simulink model "DriveSystemControl"  (R2023b)
settings: Solver=FixedStepAuto  StartTime=0.0  StopTime=Inf  FixedStep=0.001  RelTol=1e-3
PostLoadFcn:
  | if any(exist('dsrtsu_mdlpostloadfcn', 'file') ~= 0), dsrtsu_mdlpostloadfcn('Execute', bdroot); end
InitFcn:
  | , if any(exist('rtifpga_mdlclblib', 'file') ~= 0), rtifpga_mdlclblib('Init', bdroot); end,
  | , if any(exist('dsmpb_private', 'file') ~= 0), dsmpb_private('dsmpb_mdlclblib', 'Init', bdroot); end,
libraries: dsmpblib x2
(part 3 of 11)

== system DriveSystemControl/Bus Configuration (1) - In/Manipulation/Virya Controller CAN File 08082024/WIP/CANChannel/PDUs/MainController/notUsed ==
  Feature Switch : Subsystem
  ISignal Overwrite Value : Subsystem
  _notUsed_ : BusCreator  Inputs=2
  notUsed : Outport
  wires:
  _notUsed_/1 -> notUsed/1  "notUsed"
  Feature Switch/1(Feature Switch) -> _notUsed_/1  "Feature Switch"
  ISignal Overwrite Value/1(ISignal Overwrite Value) -> _notUsed_/2  "ISignal Overwrite Value"

== system DriveSystemControl/Bus Configuration (1) - In/Manipulation/Virya Controller CAN File 08082024/WIP/CANChannel/PDUs/MainController/setAutoParkBreak ==
  Feature Switch : Subsystem
  ISignal Overwrite Value : Subsystem
  _setAutoParkBreak_ : BusCreator  Inputs=2
  setAutoParkBreak : Outport
  wires:
  _setAutoParkBreak_/1 -> setAutoParkBreak/1  "setAutoParkBreak"
  Feature Switch/1(Feature Switch) -> _setAutoParkBreak_/1  "Feature Switch"
  ISignal Overwrite Value/1(ISignal Overwrite Value) -> _setAutoParkBreak_/2  "ISignal Overwrite Value"

== system DriveSystemControl/Bus Configuration (1) - In/Manipulation/Virya Controller CAN File 08082024/WIP/CANChannel/PDUs/MainController/setBreake ==
  Feature Switch : Subsystem
  ISignal Overwrite Value : Subsystem
  _setBreake_ : BusCreator  Inputs=2
  setBreake : Outport
  wires:
  _setBreake_/1 -> setBreake/1  "setBreake"
  Feature Switch/1(Feature Switch) -> _setBreake_/1  "Feature Switch"
  ISignal Overwrite Value/1(ISignal Overwrite Value) -> _setBreake_/2  "ISignal Overwrite Value"

== system DriveSystemControl/Bus Configuration (1) - In/Manipulation/Virya Controller CAN File 08082024/WIP/CANChannel/PDUs/MainController/setDirection ==
  Feature Switch : Subsystem
  ISignal Overwrite Value : Subsystem
  _setDirection_ : BusCreator  Inputs=2
  setDirection : Outport
  wires:
  _setDirection_/1 -> setDirection/1  "setDirection"
  Feature Switch/1(Feature Switch) -> _setDirection_/1  "Feature Switch"
  ISignal Overwrite Value/1(ISignal Overwrite Value) -> _setDirection_/2  "ISignal Overwrite Value"

== system DriveSystemControl/Bus Configuration (1) - In/Manipulation/Virya Controller CAN File 08082024/WIP/CANChannel/PDUs/MainController/setDriveMode ==
  Feature Switch : Subsystem
  ISignal Overwrite Value : Subsystem
  _setDriveMode_ : BusCreator  Inputs=2
  setDriveMode : Outport
  wires:
  _setDriveMode_/1 -> setDriveMode/1  "setDriveMode"
  Feature Switch/1(Feature Switch) -> _setDriveMode_/1  "Feature Switch"
  ISignal Overwrite Value/1(ISignal Overwrite Value) -> _setDriveMode_/2  "ISignal Overwrite Value"

== system DriveSystemControl/Bus Configuration (1) - In/Manipulation/Virya Controller CAN File 08082024/WIP/CANChannel/PDUs/MainController/setVelocity ==
  Feature Switch : Subsystem
  ISignal Overwrite Value : Subsystem
  _setVelocity_ : BusCreator  Inputs=2
  setVelocity : Outport
  wires:
  _setVelocity_/1 -> setVelocity/1  "setVelocity"
  Feature Switch/1(Feature Switch) -> _setVelocity_/1  "Feature Switch"
  ISignal Overwrite Value/1(ISignal Overwrite Value) -> _setVelocity_/2  "ISignal Overwrite Value"

== system DriveSystemControl/Bus Configuration (1) - In/Manipulation/Virya Controller CAN File 08082024/WIP/CANChannel/PDUs/MainController/steeringPower ==
  Feature Switch : Subsystem
  ISignal Overwrite Value : Subsystem
  _steeringPower_ : BusCreator  Inputs=2
  steeringPower : Outport
  wires:
  _steeringPower_/1 -> steeringPower/1  "steeringPower"
  Feature Switch/1(Feature Switch) -> _steeringPower_/1  "Feature Switch"
  ISignal Overwrite Value/1(ISignal Overwrite Value) -> _steeringPower_/2  "ISignal Overwrite Value"

== system DriveSystemControl/Bus Configuration (1) - In/Manipulation/Virya Controller CAN File 08082024/WIP/CANChannel/PDUs/TCU01/sigBrake ==
  Feature Switch : Subsystem
  ISignal Overwrite Value : Subsystem
  _sigBrake_ : BusCreator  Inputs=2
  sigBrake : Outport
  wires:
  _sigBrake_/1 -> sigBrake/1  "sigBrake"
  Feature Switch/1(Feature Switch) -> _sigBrake_/1  "Feature Switch"
  ISignal Overwrite Value/1(ISignal Overwrite Value) -> _sigBrake_/2  "ISignal Overwrite Value"

== system DriveSystemControl/Bus Configuration (1) - In/Manipulation/Virya Controller CAN File 08082024/WIP/CANChannel/PDUs/TCU01/sigControllerTemperature ==
  Feature Switch : Subsystem
  ISignal Overwrite Value : Subsystem
  _sigControllerTemperature_ : BusCreator  Inputs=2
  sigControllerTemperature : Outport
  wires:
  _sigControllerTemperature_/1 -> sigControllerTemperature/1  "sigControllerTemperature"
  Feature Switch/1(Feature Switch) -> _sigControllerTemperature_/1  "Feature Switch"
  ISignal Overwrite Value/1(ISignal Overwrite Value) -> _sigControllerTemperature_/2  "ISignal Overwrite Value"

== system DriveSystemControl/Bus Configuration (1) - In/Manipulation/Virya Controller CAN File 08082024/WIP/CANChannel/PDUs/TCU01/sigDriveMode ==
  Feature Switch : Subsystem
  ISignal Overwrite Value : Subsystem
  _sigDriveMode_ : BusCreator  Inputs=2
  sigDriveMode : Outport
  wires:
  _sigDriveMode_/1 -> sigDriveMode/1  "sigDriveMode"
  Feature Switch/1(Feature Switch) -> _sigDriveMode_/1  "Feature Switch"
  ISignal Overwrite Value/1(ISignal Overwrite Value) -> _sigDriveMode_/2  "ISignal Overwrite Value"

== system DriveSystemControl/Bus Configuration (1) - In/Manipulation/Virya Controller CAN File 08082024/WIP/CANChannel/PDUs/TCU01/sigMotorTemperature ==
  Feature Switch : Subsystem
  ISignal Overwrite Value : Subsystem
  _sigMotorTemperature_ : BusCreator  Inputs=2
  sigMotorTemperature : Outport
  wires:
  _sigMotorTemperature_/1 -> sigMotorTemperature/1  "sigMotorTemperature"
  Feature Switch/1(Feature Switch) -> _sigMotorTemperature_/1  "Feature Switch"
  ISignal Overwrite Value/1(ISignal Overwrite Value) -> _sigMotorTemperature_/2  "ISignal Overwrite Value"

== system DriveSystemControl/Bus Configuration (1) - In/Manipulation/Virya Controller CAN File 08082024/WIP/CANChannel/PDUs/TCU01/sigRMSCurrent ==
  Feature Switch : Subsystem
  ISignal Overwrite Value : Subsystem
  _sigRMSCurrent_ : BusCreator  Inputs=2
  sigRMSCurrent : Outport
  wires:
  _sigRMSCurrent_/1 -> sigRMSCurrent/1  "sigRMSCurrent"
  Feature Switch/1(Feature Switch) -> _sigRMSCurrent_/1  "Feature Switch"
  ISignal Overwrite Value/1(ISignal Overwrite Value) -> _sigRMSCurrent_/2  "ISignal Overwrite Value"

== system DriveSystemControl/Bus Configuration (1) - In/Manipulation/Virya Controller CAN File 08082024/WIP/CANChannel/PDUs/TCU01/sigSpeed ==
  Feature Switch : Subsystem
  ISignal Overwrite Value : Subsystem
  _sigSpeed_ : BusCreator  Inputs=2
  sigSpeed : Outport
  wires:
  _sigSpeed_/1 -> sigSpeed/1  "sigSpeed"
  Feature Switch/1(Feature Switch) -> _sigSpeed_/1  "Feature Switch"
  ISignal Overwrite Value/1(ISignal Overwrite Value) -> _sigSpeed_/2  "ISignal Overwrite Value"

== system DriveSystemControl/Bus Configuration (1) - In/Manipulation/Virya Controller CAN File 08082024/WIP/CANChannel/PDUs/TCU01/sigThrottle ==
  Feature Switch : Subsystem
  ISignal Overwrite Value : Subsystem
  _sigThrottle_ : BusCreator  Inputs=2
  sigThrottle : Outport
  wires:
  _sigThrottle_/1 -> sigThrottle/1  "sigThrottle"
  Feature Switch/1(Feature Switch) -> _sigThrottle_/1  "Feature Switch"
  ISignal Overwrite Value/1(ISignal Overwrite Value) -> _sigThrottle_/2  "ISignal Overwrite Value"

== system DriveSystemControl/Bus Configuration (1) - In/Manipulation/Virya Controller CAN File 08082024/WIP/CANChannel/PDUs/TCU02/sigCapacitorVoltage ==
  Feature Switch : Subsystem
  ISignal Overwrite Value : Subsystem
  _sigCapacitorVoltage_ : BusCreator  Inputs=2
  sigCapacitorVoltage : Outport
  wires:
  _sigCapacitorVoltage_/1 -> sigCapacitorVoltage/1  "sigCapacitorVoltage"
  Feature Switch/1(Feature Switch) -> _sigCapacitorVoltage_/1  "Feature Switch"
  ISignal Overwrite Value/1(ISignal Overwrite Value) -> _sigCapacitorVoltage_/2  "ISignal Overwrite Value"

== system DriveSystemControl/Bus Configuration (1) - In/Manipulation/Virya Controller CAN File 08082024/WIP/CANChannel/PDUs/TCU02/sigMotorRPM ==
  Feature Switch : Subsystem
  ISignal Overwrite Value : Subsystem
  _sigMotorRPM_ : BusCreator  Inputs=2
  sigMotorRPM : Outport
  wires:
  _sigMotorRPM_/1 -> sigMotorRPM/1  "sigMotorRPM"
  Feature Switch/1(Feature Switch) -> _sigMotorRPM_/1  "Feature Switch"
  ISignal Overwrite Value/1(ISignal Overwrite Value) -> _sigMotorRPM_/2  "ISignal Overwrite Value"

== system DriveSystemControl/Bus Configuration (1) - In/Manipulation/Virya Controller CAN File 08082024/WIP/CANChannel/PDUs/TCU02/sigOdometer ==
  Feature Switch : Subsystem
  ISignal Overwrite Value : Subsystem
  _sigOdometer_ : BusCreator  Inputs=2
  sigOdometer : Outport
  wires:
  _sigOdometer_/1 -> sigOdometer/1  "sigOdometer"
  Feature Switch/1(Feature Switch) -> _sigOdometer_/1  "Feature Switch"
  ISignal Overwrite Value/1(ISignal Overwrite Value) -> _sigOdometer_/2  "ISignal Overwrite Value"

== system DriveSystemControl/Bus Configuration (1) - In/Manipulation/Virya Controller CAN File 08082024/WIP/CANChannel/PDUs/TCU03/Controller_CompleteFaults ==
  Feature Switch : Subsystem
  ISignal Overwrite Value : Subsystem
  _Controller_CompleteFaults_ : BusCreator  Inputs=2
  Controller_CompleteFaults : Outport
  wires:
  _Controller_CompleteFaults_/1 -> Controller_CompleteFaults/1  "Controller_CompleteFaults"
  Feature Switch/1(Feature Switch) -> _Controller_CompleteFaults_/1  "Feature Switch"
  ISignal Overwrite Value/1(ISignal Overwrite Value) -> _Controller_CompleteFaults_/2  "ISignal Overwrite Value"

== system DriveSystemControl/Bus Configuration (1) - In/Manipulation/Virya Controller CAN File 08082024/WIP/CANChannel/PDUs/TCU03/sig5VSupplyFailure ==
  Feature Switch : Subsystem
  ISignal Overwrite Value : Subsystem
  _sig5VSupplyFailure_ : BusCreator  Inputs=2
  sig5VSupplyFailure : Outport
  wires:
  _sig5VSupplyFailure_/1 -> sig5VSupplyFailure/1  "sig5VSupplyFailure"
  Feature Switch/1(Feature Switch) -> _sig5VSupplyFailure_/1  "Feature Switch"
  ISignal Overwrite Value/1(ISignal Overwrite Value) -> _sig5VSupplyFailure_/2  "ISignal Overwrite Value"

== system DriveSystemControl/Bus Configuration (1) - In/Manipulation/Virya Controller CAN File 08082024/WIP/CANChannel/PDUs/TCU03/sigBPosOvervoltageCutback ==
  Feature Switch : Subsystem
  ISignal Overwrite Value : Subsystem
  _sigBPosOvervoltageCutback_ : BusCreator  Inputs=2
  sigBPosOvervoltageCutback : Outport
  wires:
  _sigBPosOvervoltageCutback_/1 -> sigBPosOvervoltageCutback/1  "sigBPosOvervoltageCutback"
  Feature Switch/1(Feature Switch) -> _sigBPosOvervoltageCutback_/1  "Feature Switch"
  ISignal Overwrite Value/1(ISignal Overwrite Value) -> _sigBPosOvervoltageCutback_/2  "ISignal Overwrite Value"

== system DriveSystemControl/Bus Configuration (1) - In/Manipulation/Virya Controller CAN File 08082024/WIP/CANChannel/PDUs/TCU03/sigBPosUndervoltageCutback ==
  Feature Switch : Subsystem
  ISignal Overwrite Value : Subsystem
  _sigBPosUndervoltageCutback_ : BusCreator  Inputs=2
  sigBPosUndervoltageCutback : Outport
  wires:
  _sigBPosUndervoltageCutback_/1 -> sigBPosUndervoltageCutback/1  "sigBPosUndervoltageCutback"
  Feature Switch/1(Feature Switch) -> _sigBPosUndervoltageCutback_/1  "Feature Switch"
  ISignal Overwrite Value/1(ISignal Overwrite Value) -> _sigBPosUndervoltageCutback_/2  "ISignal Overwrite Value"

== system DriveSystemControl/Bus Configuration (1) - In/Manipulation/Virya Controller CAN File 08082024/WIP/CANChannel/PDUs/TCU03/sigBadCalibration ==
  Feature Switch : Subsystem
  ISignal Overwrite Value : Subsystem
  _sigBadCalibration_ : BusCreator  Inputs=2
  sigBadCalibration : Outport
  wires:
  _sigBadCalibration_/1 -> sigBadCalibration/1  "sigBadCalibration"
  Feature Switch/1(Feature Switch) -> _sigBadCalibration_/1  "Feature Switch"
  ISignal Overwrite Value/1(ISignal Overwrite Value) -> _sigBadCalibration_/2  "ISignal Overwrite Value"

== system DriveSystemControl/Bus Configuration (1) - In/Manipulation/Virya Controller CAN File 08082024/WIP/CANChannel/PDUs/TCU03/sigBrakeWiperHigh ==
  Feature Switch : Subsystem
  ISignal Overwrite Value : Subsystem
  _sigBrakeWiperHigh_ : BusCreator  Inputs=2
  sigBrakeWiperHigh : Outport
  wires:
  _sigBrakeWiperHigh_/1 -> sigBrakeWiperHigh/1  "sigBrakeWiperHigh"
  Feature Switch/1(Feature Switch) -> _sigBrakeWiperHigh_/1  "Feature Switch"
  ISignal Overwrite Value/1(ISignal Overwrite Value) -> _sigBrakeWiperHigh_/2  "ISignal Overwrite Value"

== system DriveSystemControl/Bus Configuration (1) - In/Manipulation/Virya Controller CAN File 08082024/WIP/CANChannel/PDUs/TCU03/sigBrakeWiperLow ==
  Feature Switch : Subsystem
  ISignal Overwrite Value : Subsystem
  _sigBrakeWiperLow_ : BusCreator  Inputs=2
  sigBrakeWiperLow : Outport
  wires:
  _sigBrakeWiperLow_/1 -> sigBrakeWiperLow/1  "sigBrakeWiperLow"
  Feature Switch/1(Feature Switch) -> _sigBrakeWiperLow_/1  "Feature Switch"
  ISignal Overwrite Value/1(ISignal Overwrite Value) -> _sigBrakeWiperLow_/2  "ISignal Overwrite Value"

== system DriveSystemControl/Bus Configuration (1) - In/Manipulation/Virya Controller CAN File 08082024/WIP/CANChannel/PDUs/TCU03/sigCoil2DriverOpenShort ==
  Feature Switch : Subsystem
  ISignal Overwrite Value : Subsystem
  _sigCoil2DriverOpenShort_ : BusCreator  Inputs=2
  sigCoil2DriverOpenShort : Outport
  wires:
  _sigCoil2DriverOpenShort_/1 -> sigCoil2DriverOpenShort/1  "sigCoil2DriverOpenShort"
  Feature Switch/1(Feature Switch) -> _sigCoil2DriverOpenShort_/1  "Feature Switch"
  ISignal Overwrite Value/1(ISignal Overwrite Value) -> _sigCoil2DriverOpenShort_/2  "ISignal Overwrite Value"

== system DriveSystemControl/Bus Configuration (1) - In/Manipulation/Virya Controller CAN File 08082024/WIP/CANChannel/PDUs/TCU03/sigCoil3DriverOpenShort ==
  Feature Switch : Subsystem
  ISignal Overwrite Value : Subsystem
  _sigCoil3DriverOpenShort_ : BusCreator  Inputs=2
  sigCoil3DriverOpenShort : Outport
  wires:
  _sigCoil3DriverOpenShort_/1 -> sigCoil3DriverOpenShort/1  "sigCoil3DriverOpenShort"
  Feature Switch/1(Feature Switch) -> _sigCoil3DriverOpenShort_/1  "Feature Switch"
  ISignal Overwrite Value/1(ISignal Overwrite Value) -> _sigCoil3DriverOpenShort_/2  "ISignal Overwrite Value"

== system DriveSystemControl/Bus Configuration (1) - In/Manipulation/Virya Controller CAN File 08082024/WIP/CANChannel/PDUs/TCU03/sigCoil4DriverOpenShort ==
  Feature Switch : Subsystem
  ISignal Overwrite Value : Subsystem
  _sigCoil4DriverOpenShort_ : BusCreator  Inputs=2
  sigCoil4DriverOpenShort : Outport
  wires:
  _sigCoil4DriverOpenShort_/1 -> sigCoil4DriverOpenShort/1  "sigCoil4DriverOpenShort"
  Feature Switch/1(Feature Switch) -> _sigCoil4DriverOpenShort_/1  "Feature Switch"
  ISignal Overwrite Value/1(ISignal Overwrite Value) -> _sigCoil4DriverOpenShort_/2  "ISignal Overwrite Value"

== system DriveSystemControl/Bus Configuration (1) - In/Manipulation/Virya Controller CAN File 08082024/WIP/CANChannel/PDUs/TCU03/sigControllerCommonFault ==
  Feature Switch : Subsystem
  ISignal Overwrite Value : Subsystem
  _sigControllerCommonFault_ : BusCreator  Inputs=2
  sigControllerCommonFault : Outport
  wires:
  _sigControllerCommonFault_/1 -> sigControllerCommonFault/1  "sigControllerCommonFault"
  Feature Switch/1(Feature Switch) -> _sigControllerCommonFault_/1  "Feature Switch"
  ISignal Overwrite Value/1(ISignal Overwrite Value) -> _sigControllerCommonFault_/2  "ISignal Overwrite Value"

== system DriveSystemControl/Bus Configuration (1) - In/Manipulation/Virya Controller CAN File 08082024/WIP/CANChannel/PDUs/TCU03/sigControllerOverCurrent ==
  Feature Switch : Subsystem
  ISignal Overwrite Value : Subsystem
  _sigControllerOverCurrent_ : BusCreator  Inputs=2
  sigControllerOverCurrent : Outport
  wires:
  _sigControllerOverCurrent_/1 -> sigControllerOverCurrent/1  "sigControllerOverCurrent"
  Feature Switch/1(Feature Switch) -> _sigControllerOverCurrent_/1  "Feature Switch"
  ISignal Overwrite Value/1(ISignal Overwrite Value) -> _sigControllerOverCurrent_/2  "ISignal Overwrite Value"

== system DriveSystemControl/Bus Configuration (1) - In/Manipulation/Virya Controller CAN File 08082024/WIP/CANChannel/PDUs/TCU03/sigControllerOvertempCutback ==
  Feature Switch : Subsystem
  ISignal Overwrite Value : Subsystem
  _sigControllerOvertempCutback_ : BusCreator  Inputs=2
  sigControllerOvertempCutback : Outport
  wires:
  _sigControllerOvertempCutback_/1 -> sigControllerOvertempCutback/1  "sigControllerOvertempCutback"
  Feature Switch/1(Feature Switch) -> _sigControllerOvertempCutback_/1  "Feature Switch"
  ISignal Overwrite Value/1(ISignal Overwrite Value) -> _sigControllerOvertempCutback_/2  "ISignal Overwrite Value"

== system DriveSystemControl/Bus Configuration (1) - In/Manipulation/Virya Controller CAN File 08082024/WIP/CANChannel/PDUs/TCU03/sigControllerSevereOvertemp ==
  Feature Switch : Subsystem
  ISignal Overwrite Value : Subsystem
  _sigControllerSevereOvertemp_ : BusCreator  Inputs=2
  sigControllerSevereOvertemp : Outport
  wires:
  _sigControllerSevereOvertemp_/1 -> sigControllerSevereOvertemp/1  "sigControllerSevereOvertemp"
  Feature Switch/1(Feature Switch) -> _sigControllerSevereOvertemp_/1  "Feature Switch"
  ISignal Overwrite Value/1(ISignal Overwrite Value) -> _sigControllerSevereOvertemp_/2  "ISignal Overwrite Value"

== system DriveSystemControl/Bus Configuration (1) - In/Manipulation/Virya Controller CAN File 08082024/WIP/CANChannel/PDUs/TCU03/sigControllerSevereUndertemp ==
  Feature Switch : Subsystem
  ISignal Overwrite Value : Subsystem
  _sigControllerSevereUndertemp_ : BusCreator  Inputs=2
  sigControllerSevereUndertemp : Outport
  wires:
  _sigControllerSevereUndertemp_/1 -> sigControllerSevereUndertemp/1  "sigControllerSevereUndertemp"
  Feature Switch/1(Feature Switch) -> _sigControllerSevereUndertemp_/1  "Feature Switch"
  ISignal Overwrite Value/1(ISignal Overwrite Value) -> _sigControllerSevereUndertemp_/2  "ISignal Overwrite Value"

== system DriveSystemControl/Bus Configuration (1) - In/Manipulation/Virya Controller CAN File 08082024/WIP/CANChannel/PDUs/TCU03/sigCurrentSensorFault ==
  Feature Switch : Subsystem
  ISignal Overwrite Value : Subsystem
  _sigCurrentSensorFault_ : BusCreator  Inputs=2
  sigCurrentSensorFault : Outport
  wires:
  _sigCurrentSensorFault_/1 -> sigCurrentSensorFault/1  "sigCurrentSensorFault"
  Feature Switch/1(Feature Switch) -> _sigCurrentSensorFault_/1  "Feature Switch"
  ISignal Overwrite Value/1(ISignal Overwrite Value) -> _sigCurrentSensorFault_/2  "ISignal Overwrite Value"

== system DriveSystemControl/Bus Configuration (1) - In/Manipulation/Virya Controller CAN File 08082024/WIP/CANChannel/PDUs/TCU03/sigEEPROMFailure ==
  Feature Switch : Subsystem
  ISignal Overwrite Value : Subsystem
  _sigEEPROMFailure_ : BusCreator  Inputs=2
  sigEEPROMFailure : Outport
  wires:
  _sigEEPROMFailure_/1 -> sigEEPROMFailure/1  "sigEEPROMFailure"
  Feature Switch/1(Feature Switch) -> _sigEEPROMFailure_/1  "Feature Switch"
  ISignal Overwrite Value/1(ISignal Overwrite Value) -> _sigEEPROMFailure_/2  "ISignal Overwrite Value"

== system DriveSystemControl/Bus Configuration (1) - In/Manipulation/Virya Controller CAN File 08082024/WIP/CANChannel/PDUs/TCU03/sigHighPedalDisable ==
  Feature Switch : Subsystem
  ISignal Overwrite Value : Subsystem
  _sigHighPedalDisable_ : BusCreator  Inputs=2
  sigHighPedalDisable : Outport
  wires:
  _sigHighPedalDisable_/1 -> sigHighPedalDisable/1  "sigHighPedalDisable"
  Feature Switch/1(Feature Switch) -> _sigHighPedalDisable_/1  "Feature Switch"
  ISignal Overwrite Value/1(ISignal Overwrite Value) -> _sigHighPedalDisable_/2  "ISignal Overwrite Value"

== system DriveSystemControl/Bus Configuration (1) - In/Manipulation/Virya Controller CAN File 08082024/WIP/CANChannel/PDUs/TCU03/sigInsulationResistanceLow ==
  Feature Switch : Subsystem
  ISignal Overwrite Value : Subsystem
  _sigInsulationResistanceLow_ : BusCreator  Inputs=2
  sigInsulationResistanceLow : Outport
  wires:
  _sigInsulationResistanceLow_/1 -> sigInsulationResistanceLow/1  "sigInsulationResistanceLow"
  Feature Switch/1(Feature Switch) -> _sigInsulationResistanceLow_/1  "Feature Switch"
  ISignal Overwrite Value/1(ISignal Overwrite Value) -> _sigInsulationResistanceLow_/2  "ISignal Overwrite Value"

== system DriveSystemControl/Bus Configuration (1) - In/Manipulation/Virya Controller CAN File 08082024/WIP/CANChannel/PDUs/TCU03/sigMainContactorWelded ==
  Feature Switch : Subsystem
  ISignal Overwrite Value : Subsystem
  _sigMainContactorWelded_ : BusCreator  Inputs=2
  sigMainContactorWelded : Outport
  wires:
  _sigMainContactorWelded_/1 -> sigMainContactorWelded/1  "sigMainContactorWelded"
  Feature Switch/1(Feature Switch) -> _sigMainContactorWelded_/1  "Feature Switch"
  ISignal Overwrite Value/1(ISignal Overwrite Value) -> _sigMainContactorWelded_/2  "ISignal Overwrite Value"

== system DriveSystemControl/Bus Configuration (1) - In/Manipulation/Virya Controller CAN File 08082024/WIP/CANChannel/PDUs/TCU03/sigMainContactordidnotClose ==
  Feature Switch : Subsystem
  ISignal Overwrite Value : Subsystem
  _sigMainContactordidnotClose_ : BusCreator  Inputs=2
  sigMainContactordidnotClose : Outport
  wires:
  _sigMainContactordidnotClose_/1 -> sigMainContactordidnotClose/1  "sigMainContactordidnotClose"
  Feature Switch/1(Feature Switch) -> _sigMainContactordidnotClose_/1  "Feature Switch"
  ISignal Overwrite Value/1(ISignal Overwrite Value) -> _sigMainContactordidnotClose_/2  "ISignal Overwrite Value"

== system DriveSystemControl/Bus Configuration (1) - In/Manipulation/Virya Controller CAN File 08082024/WIP/CANChannel/PDUs/TCU03/sigMainOpenShort ==
  Feature Switch : Subsystem
  ISignal Overwrite Value : Subsystem
  _sigMainOpenShort_ : BusCreator  Inputs=2
  sigMainOpenShort : Outport
  wires:
  _sigMainOpenShort_/1 -> sigMainOpenShort/1  "sigMainOpenShort"
  Feature Switch/1(Feature Switch) -> _sigMainOpenShort_/1  "Feature Switch"
  ISignal Overwrite Value/1(ISignal Overwrite Value) -> _sigMainOpenShort_/2  "ISignal Overwrite Value"

== system DriveSystemControl/Bus Configuration (1) - In/Manipulation/Virya Controller CAN File 08082024/WIP/CANChannel/PDUs/TCU03/sigMotorCharacterization ==
  Feature Switch : Subsystem
  ISignal Overwrite Value : Subsystem
  _sigMotorCharacterization_ : BusCreator  Inputs=2
  sigMotorCharacterization : Outport
  wires:
  _sigMotorCharacterization_/1 -> sigMotorCharacterization/1  "sigMotorCharacterization"
  Feature Switch/1(Feature Switch) -> _sigMotorCharacterization_/1  "Feature Switch"
  ISignal Overwrite Value/1(ISignal Overwrite Value) -> _sigMotorCharacterization_/2  "ISignal Overwrite Value"

== system DriveSystemControl/Bus Configuration (1) - In/Manipulation/Virya Controller CAN File 08082024/WIP/CANChannel/PDUs/TCU03/sigMotorPhaseOpen ==
  Feature Switch : Subsystem
  ISignal Overwrite Value : Subsystem
  _sigMotorPhaseOpen_ : BusCreator  Inputs=2
  sigMotorPhaseOpen : Outport
  wires:
  _sigMotorPhaseOpen_/1 -> sigMotorPhaseOpen/1  "sigMotorPhaseOpen"
  Feature Switch/1(Feature Switch) -> _sigMotorPhaseOpen_/1  "Feature Switch"
  ISignal Overwrite Value/1(ISignal Overwrite Value) -> _sigMotorPhaseOpen_/2  "ISignal Overwrite Value"

== system DriveSystemControl/Bus Configuration (1) - In/Manipulation/Virya Controller CAN File 08082024/WIP/CANChannel/PDUs/TCU03/sigMotorTempHotCutback ==
  Feature Switch : Subsystem
  ISignal Overwrite Value : Subsystem
  _sigMotorTempHotCutback_ : BusCreator  Inputs=2
  sigMotorTempHotCutback : Outport
  wires:
  _sigMotorTempHotCutback_/1 -> sigMotorTempHotCutback/1  "sigMotorTempHotCutback"
  Feature Switch/1(Feature Switch) -> _sigMotorTempHotCutback_/1  "Feature Switch"
  ISignal Overwrite Value/1(ISignal Overwrite Value) -> _sigMotorTempHotCutback_/2  "ISignal Overwrite Value"

== system DriveSystemControl/Bus Configuration (1) - In/Manipulation/Virya Controller CAN File 08082024/WIP/CANChannel/PDUs/TCU03/sigMotorTempSensorFault ==
  Feature Switch : Subsystem
  ISignal Overwrite Value : Subsystem
  _sigMotorTempSensorFault_ : BusCreator  Inputs=2
  sigMotorTempSensorFault : Outport
  wires:
  _sigMotorTempSensorFault_/1 -> sigMotorTempSensorFault/1  "sigMotorTempSensorFault"
  Feature Switch/1(Feature Switch) -> _sigMotorTempSensorFault_/1  "Feature Switch"
  ISignal Overwrite Value/1(ISignal Overwrite Value) -> _sigMotorTempSensorFault_/2  "ISignal Overwrite Value"

== system DriveSystemControl/Bus Configuration (1) - In/Manipulation/Virya Controller CAN File 08082024/WIP/CANChannel/PDUs/TCU03/sigOEM_BatterySTOPSignal ==
  Feature Switch : Subsystem
  ISignal Overwrite Value : Subsystem
  _sigOEM_BatterySTOPSignal_ : BusCreator  Inputs=2
  sigOEM_BatterySTOPSignal : Outport
  wires:
  _sigOEM_BatterySTOPSignal_/1 -> sigOEM_BatterySTOPSignal/1  "sigOEM_BatterySTOPSignal"
  Feature Switch/1(Feature Switch) -> _sigOEM_BatterySTOPSignal_/1  "Feature Switch"
  ISignal Overwrite Value/1(ISignal Overwrite Value) -> _sigOEM_BatterySTOPSignal_/2  "ISignal Overwrite Value"

== system DriveSystemControl/Bus Configuration (1) - In/Manipulation/Virya Controller CAN File 08082024/WIP/CANChannel/PDUs/TCU03/sigOEM_NoBatteryCAN ==
  Feature Switch : Subsystem
  ISignal Overwrite Value : Subsystem
  _sigOEM_NoBatteryCAN_ : BusCreator  Inputs=2
  sigOEM_NoBatteryCAN : Outport
  wires:
  _sigOEM_NoBatteryCAN_/1 -> sigOEM_NoBatteryCAN/1  "sigOEM_NoBatteryCAN"
  Feature Switch/1(Feature Switch) -> _sigOEM_NoBatteryCAN_/1  "Feature Switch"
  ISignal Overwrite Value/1(ISignal Overwrite Value) -> _sigOEM_NoBatteryCAN_/2  "ISignal Overwrite Value"

== system DriveSystemControl/Bus Configuration (1) - In/Manipulation/Virya Controller CAN File 08082024/WIP/CANChannel/PDUs/TCU03/sigOSGeneral ==
  Feature Switch : Subsystem
  ISignal Overwrite Value : Subsystem
  _sigOSGeneral_ : BusCreator  Inputs=2
  sigOSGeneral : Outport
  wires:
  _sigOSGeneral_/1 -> sigOSGeneral/1  "sigOSGeneral"
  Feature Switch/1(Feature Switch) -> _sigOSGeneral_/1  "Feature Switch"
  ISignal Overwrite Value/1(ISignal Overwrite Value) -> _sigOSGeneral_/2  "ISignal Overwrite Value"

== system DriveSystemControl/Bus Configuration (1) - In/Manipulation/Virya Controller CAN File 08082024/WIP/CANChannel/PDUs/TCU03/sigPMACCommissioningNeeded ==
  Feature Switch : Subsystem
  ISignal Overwrite Value : Subsystem
  _sigPMACCommissioningNeeded_ : BusCreator  Inputs=2
  sigPMACCommissioningNeeded : Outport
  wires:
  _sigPMACCommissioningNeeded_/1 -> sigPMACCommissioningNeeded/1  "sigPMACCommissioningNeeded"
  Feature Switch/1(Feature Switch) -> _sigPMACCommissioningNeeded_/1  "Feature Switch"
  ISignal Overwrite Value/1(ISignal Overwrite Value) -> _sigPMACCommissioningNeeded_/2  "ISignal Overwrite Value"

== system DriveSystemControl/Bus Configuration (1) - In/Manipulation/Virya Controller CAN File 08082024/WIP/CANChannel/PDUs/TCU03/sigParameterChangeFault ==
  Feature Switch : Subsystem
  ISignal Overwrite Value : Subsystem
  _sigParameterChangeFault_ : BusCreator  Inputs=2
  sigParameterChangeFault : Outport
  wires:
  _sigParameterChangeFault_/1 -> sigParameterChangeFault/1  "sigParameterChangeFault"
  Feature Switch/1(Feature Switch) -> _sigParameterChangeFault_/1  "Feature Switch"
  ISignal Overwrite Value/1(ISignal Overwrite Value) -> _sigParameterChangeFault_/2  "ISignal Overwrite Value"

== system DriveSystemControl/Bus Configuration (1) - In/Manipulation/Virya Controller CAN File 08082024/WIP/CANChannel/PDUs/TCU03/sigPhasePWMMismatch ==
  Feature Switch : Subsystem
  ISignal Overwrite Value : Subsystem
  _sigPhasePWMMismatch_ : BusCreator  Inputs=2
  sigPhasePWMMismatch : Outport
  wires:
  _sigPhasePWMMismatch_/1 -> sigPhasePWMMismatch/1  "sigPhasePWMMismatch"
  Feature Switch/1(Feature Switch) -> _sigPhasePWMMismatch_/1  "Feature Switch"
  ISignal Overwrite Value/1(ISignal Overwrite Value) -> _sigPhasePWMMismatch_/2  "ISignal Overwrite Value"

== system DriveSystemControl/Bus Configuration (1) - In/Manipulation/Virya Controller CAN File 08082024/WIP/CANChannel/PDUs/TCU03/sigPrechargeFailed ==
  Feature Switch : Subsystem
  ISignal Overwrite Value : Subsystem
  _sigPrechargeFailed_ : BusCreator  Inputs=2
  sigPrechargeFailed : Outport
  wires:
  _sigPrechargeFailed_/1 -> sigPrechargeFailed/1  "sigPrechargeFailed"
  Feature Switch/1(Feature Switch) -> _sigPrechargeFailed_/1  "Feature Switch"
  ISignal Overwrite Value/1(ISignal Overwrite Value) -> _sigPrechargeFailed_/2  "ISignal Overwrite Value"

== system DriveSystemControl/Bus Configuration (1) - In/Manipulation/Virya Controller CAN File 08082024/WIP/CANChannel/PDUs/TCU03/sigSevereBPosOvervoltage ==
  Feature Switch : Subsystem
  ISignal Overwrite Value : Subsystem
  _sigSevereBPosOvervoltage_ : BusCreator  Inputs=2
  sigSevereBPosOvervoltage : Outport
  wires:
  _sigSevereBPosOvervoltage_/1 -> sigSevereBPosOvervoltage/1  "sigSevereBPosOvervoltage"
  Feature Switch/1(Feature Switch) -> _sigSevereBPosOvervoltage_/1  "Feature Switch"
  ISignal Overwrite Value/1(ISignal Overwrite Value) -> _sigSevereBPosOvervoltage_/2  "ISignal Overwrite Value"

== system DriveSystemControl/Bus Configuration (1) - In/Manipulation/Virya Controller CAN File 08082024/WIP/CANChannel/PDUs/TCU03/sigSevereBPosUndervoltage ==
  Feature Switch : Subsystem
  ISignal Overwrite Value : Subsystem
  _sigSevereBPosUndervoltage_ : BusCreator  Inputs=2
  sigSevereBPosUndervoltage : Outport
  wires:
  _sigSevereBPosUndervoltage_/1 -> sigSevereBPosUndervoltage/1  "sigSevereBPosUndervoltage"
  Feature Switch/1(Feature Switch) -> _sigSevereBPosUndervoltage_/1  "Feature Switch"
  ISignal Overwrite Value/1(ISignal Overwrite Value) -> _sigSevereBPosUndervoltage_/2  "ISignal Overwrite Value"

== system DriveSystemControl/Bus Configuration (1) - In/Manipulation/Virya Controller CAN File 08082024/WIP/CANChannel/PDUs/TCU03/sigSevereKSIOvervoltage ==
  Feature Switch : Subsystem
  ISignal Overwrite Value : Subsystem
  _sigSevereKSIOvervoltage_ : BusCreator  Inputs=2
  sigSevereKSIOvervoltage : Outport
  wires:
  _sigSevereKSIOvervoltage_/1 -> sigSevereKSIOvervoltage/1  "sigSevereKSIOvervoltage"
  Feature Switch/1(Feature Switch) -> _sigSevereKSIOvervoltage_/1  "Feature Switch"
  ISignal Overwrite Value/1(ISignal Overwrite Value) -> _sigSevereKSIOvervoltage_/2  "ISignal Overwrite Value"

== system DriveSystemControl/Bus Configuration (1) - In/Manipulation/Virya Controller CAN File 08082024/WIP/CANChannel/PDUs/TCU03/sigSevereKSIUndervoltage ==
  Feature Switch : Subsystem
  ISignal Overwrite Value : Subsystem
  _sigSevereKSIUndervoltage_ : BusCreator  Inputs=2
  sigSevereKSIUndervoltage : Outport
  wires:
  _sigSevereKSIUndervoltage_/1 -> sigSevereKSIUndervoltage/1  "sigSevereKSIUndervoltage"
  Feature Switch/1(Feature Switch) -> _sigSevereKSIUndervoltage_/1  "Feature Switch"
  ISignal Overwrite Value/1(ISignal Overwrite Value) -> _sigSevereKSIUndervoltage_/2  "ISignal Overwrite Value"

== system DriveSystemControl/Bus Configuration (1) - In/Manipulation/Virya Controller CAN File 08082024/WIP/CANChannel/PDUs/TCU03/sigSinCosMisalignment ==
  Feature Switch : Subsystem
  ISignal Overwrite Value : Subsystem
  _sigSinCosMisalignment_ : BusCreator  Inputs=2
  sigSinCosMisalignment : Outport
  wires:
  _sigSinCosMisalignment_/1 -> sigSinCosMisalignment/1  "sigSinCosMisalignment"
  Feature Switch/1(Feature Switch) -> _sigSinCosMisalignment_/1  "Feature Switch"
  ISignal Overwrite Value/1(ISignal Overwrite Value) -> _sigSinCosMisalignment_/2  "ISignal Overwrite Value"

== system DriveSystemControl/Bus Configuration (1) - In/Manipulation/Virya Controller CAN File 08082024/WIP/CANChannel/PDUs/TCU03/sigSinCosSensorFault ==
  Feature Switch : Subsystem
  ISignal Overwrite Value : Subsystem
  _sigSinCosSensorFault_ : BusCreator  Inputs=2
  sigSinCosSensorFault : Outport
  wires:
  _sigSinCosSensorFault_/1 -> sigSinCosSensorFault/1  "sigSinCosSensorFault"
  Feature Switch/1(Feature Switch) -> _sigSinCosSensorFault_/1  "Feature Switch"
  ISignal Overwrite Value/1(ISignal Overwrite Value) -> _sigSinCosSensorFault_/2  "ISignal Overwrite Value"

== system DriveSystemControl/Bus Configuration (1) - In/Manipulation/Virya Controller CAN File 08082024/WIP/CANChannel/PDUs/TCU03/sigStallDetected ==
  Feature Switch : Subsystem
  ISignal Overwrite Value : Subsystem
  _sigStallDetected_ : BusCreator  Inputs=2
  sigStallDetected : Outport
  wires:
  _sigStallDetected_/1 -> sigStallDetected/1  "sigStallDetected"
  Feature Switch/1(Feature Switch) -> _sigStallDetected_/1  "Feature Switch"
  ISignal Overwrite Value/1(ISignal Overwrite Value) -> _sigStallDetected_/2  "ISignal Overwrite Value"

== system DriveSystemControl/Bus Configuration (1) - In/Manipulation/Virya Controller CAN File 08082024/WIP/CANChannel/PDUs/TCU03/sigSupervisorFault ==
  Feature Switch : Subsystem
  ISignal Overwrite Value : Subsystem
  _sigSupervisorFault_ : BusCreator  Inputs=2
  sigSupervisorFault : Outport
  wires:
  _sigSupervisorFault_/1 -> sigSupervisorFault/1  "sigSupervisorFault"
  Feature Switch/1(Feature Switch) -> _sigSupervisorFault_/1  "Feature Switch"
  ISignal Overwrite Value/1(ISignal Overwrite Value) -> _sigSupervisorFault_/2  "ISignal Overwrite Value"

== system DriveSystemControl/Bus Configuration (1) - In/Manipulation/Virya Controller CAN File 08082024/WIP/CANChannel/PDUs/TCU03/sigThrottlewiperHigh ==
  Feature Switch : Subsystem
  ISignal Overwrite Value : Subsystem
  _sigThrottlewiperHigh_ : BusCreator  Inputs=2
  sigThrottlewiperHigh : Outport
  wires:
  _sigThrottlewiperHigh_/1 -> sigThrottlewiperHigh/1  "sigThrottlewiperHigh"
  Feature Switch/1(Feature Switch) -> _sigThrottlewiperHigh_/1  "Feature Switch"
  ISignal Overwrite Value/1(ISignal Overwrite Value) -> _sigThrottlewiperHigh_/2  "ISignal Overwrite Value"

== system DriveSystemControl/Bus Configuration (1) - In/Manipulation/Virya Controller CAN File 08082024/WIP/CANChannel/PDUs/TCU03/sigThrottlewiperLow ==
  Feature Switch : Subsystem
  ISignal Overwrite Value : Subsystem
  _sigThrottlewiperLow_ : BusCreator  Inputs=2
  sigThrottlewiperLow : Outport
  wires:
  _sigThrottlewiperLow_/1 -> sigThrottlewiperLow/1  "sigThrottlewiperLow"
  Feature Switch/1(Feature Switch) -> _sigThrottlewiperLow_/1  "Feature Switch"
  ISignal Overwrite Value/1(ISignal Overwrite Value) -> _sigThrottlewiperLow_/2  "ISignal Overwrite Value"

== system DriveSystemControl/Bus Configuration (1) - In/Manipulation/Virya Controller CAN File 08082024/WIP/CANChannel/PDUs/TCU03/sigVCLRunTimeError ==
  Feature Switch : Subsystem
  ISignal Overwrite Value : Subsystem
  _sigVCLRunTimeError_ : BusCreator  Inputs=2
  sigVCLRunTimeError : Outport
  wires:
  _sigVCLRunTimeError_/1 -> sigVCLRunTimeError/1  "sigVCLRunTimeError"
  Feature Switch/1(Feature Switch) -> _sigVCLRunTimeError_/1  "Feature Switch"
  ISignal Overwrite Value/1(ISignal Overwrite Value) -> _sigVCLRunTimeError_/2  "ISignal Overwrite Value"

== system DriveSystemControl/Bus Configuration (1) - In/Manipulation/Virya Controller CAN File 08082024/WIP/CANChannel/PDUs/TCU04/sigMCU5_DriveMode ==
  Feature Switch : Subsystem
  ISignal Overwrite Value : Subsystem
  _sigMCU5_DriveMode_ : BusCreator  Inputs=2
  sigMCU5_DriveMode : Outport
  wires:
  _sigMCU5_DriveMode_/1 -> sigMCU5_DriveMode/1  "sigMCU5_DriveMode"
  Feature Switch/1(Feature Switch) -> _sigMCU5_DriveMode_/1  "Feature Switch"
  ISignal Overwrite Value/1(ISignal Overwrite Value) -> _sigMCU5_DriveMode_/2  "ISignal Overwrite Value"

== system DriveSystemControl/Bus Configuration (1) - In/Manipulation/Virya Controller CAN File 08082024/WIP/CANChannel/PDUs/TCU04/sigMCU5_Efficiency ==
  Feature Switch : Subsystem
  ISignal Overwrite Value : Subsystem
  _sigMCU5_Efficiency_ : BusCreator  Inputs=2
  sigMCU5_Efficiency : Outport
  wires:
  _sigMCU5_Efficiency_/1 -> sigMCU5_Efficiency/1  "sigMCU5_Efficiency"
  Feature Switch/1(Feature Switch) -> _sigMCU5_Efficiency_/1  "Feature Switch"
  ISignal Overwrite Value/1(ISignal Overwrite Value) -> _sigMCU5_Efficiency_/2  "ISignal Overwrite Value"

== system DriveSystemControl/Bus Configuration (1) - In/Manipulation/Virya Controller CAN File 08082024/WIP/CANChannel/PDUs/TCU04/sigMCU5_Hillhold ==
  Feature Switch : Subsystem
  ISignal Overwrite Value : Subsystem
  _sigMCU5_Hillhold_ : BusCreator  Inputs=2
  sigMCU5_Hillhold : Outport
  wires:
  _sigMCU5_Hillhold_/1 -> sigMCU5_Hillhold/1  "sigMCU5_Hillhold"
  Feature Switch/1(Feature Switch) -> _sigMCU5_Hillhold_/1  "Feature Switch"
  ISignal Overwrite Value/1(ISignal Overwrite Value) -> _sigMCU5_Hillhold_/2  "ISignal Overwrite Value"

== system DriveSystemControl/Bus Configuration (1) - In/Manipulation/Virya Controller CAN File 08082024/WIP/CANChannel/PDUs/TCU04/sigMCU5_RegenFlag ==
  Feature Switch : Subsystem
  ISignal Overwrite Value : Subsystem
  _sigMCU5_RegenFlag_ : BusCreator  Inputs=2
  sigMCU5_RegenFlag : Outport
  wires:
  _sigMCU5_RegenFlag_/1 -> sigMCU5_RegenFlag/1  "sigMCU5_RegenFlag"
  Feature Switch/1(Feature Switch) -> _sigMCU5_RegenFlag_/1  "Feature Switch"
  ISignal Overwrite Value/1(ISignal Overwrite Value) -> _sigMCU5_RegenFlag_/2  "ISignal Overwrite Value"

== system DriveSystemControl/Bus Configuration (1) - In/Manipulation/Virya Controller CAN File 08082024/WIP/CANChannel/PDUs/TCU04/sigMCU5_Speed ==
  Feature Switch : Subsystem
  ISignal Overwrite Value : Subsystem
  _sigMCU5_Speed_ : BusCreator  Inputs=2
  sigMCU5_Speed : Outport
  wires:
  _sigMCU5_Speed_/1 -> sigMCU5_Speed/1  "sigMCU5_Speed"
  Feature Switch/1(Feature Switch) -> _sigMCU5_Speed_/1  "Feature Switch"
  ISignal Overwrite Value/1(ISignal Overwrite Value) -> _sigMCU5_Speed_/2  "ISignal Overwrite Value"

== system DriveSystemControl/Bus Configuration (1) - In/Manipulation/Virya Controller CAN File 08082024/WIP/CANChannel/PDUs/TCU05/sigMCU6_Odometer ==
  Feature Switch : Subsystem
  ISignal Overwrite Value : Subsystem
  _sigMCU6_Odometer_ : BusCreator  Inputs=2
  sigMCU6_Odometer : Outport
  wires:
  _sigMCU6_Odometer_/1 -> sigMCU6_Odometer/1  "sigMCU6_Odometer"
  Feature Switch/1(Feature Switch) -> _sigMCU6_Odometer_/1  "Feature Switch"
  ISignal Overwrite Value/1(ISignal Overwrite Value) -> _sigMCU6_Odometer_/2  "ISignal Overwrite Value"

== system DriveSystemControl/Bus Configuration (1) - In/Simulated ECUs/Virya Controller CAN File 08082024/BMS/TX/PDUs/BMS01/sigBatteryMalfunctionLight ==
  ISignal Value : Subsystem
  _sigBatteryMalfunctionLight_ : BusCreator  Inputs=1
  sigBatteryMalfunctionLight : Outport
  wires:
  _sigBatteryMalfunctionLight_/1 -> sigBatteryMalfunctionLight/1  "sigBatteryMalfunctionLight"
  ISignal Value/1(ISignal Value) -> _sigBatteryMalfunctionLight_/1  "ISignal Value"

== system DriveSystemControl/Bus Configuration (1) - In/Simulated ECUs/Virya Controller CAN File 08082024/BMS/TX/PDUs/BMS01/sigKeyOnIndicator ==
  ISignal Value : Subsystem
  _sigKeyOnIndicator_ : BusCreator  Inputs=1
  sigKeyOnIndicator : Outport
  wires:
  _sigKeyOnIndicator_/1 -> sigKeyOnIndicator/1  "sigKeyOnIndicator"
  ISignal Value/1(ISignal Value) -> _sigKeyOnIndicator_/1  "ISignal Value"

== system DriveSystemControl/Bus Configuration (1) - In/Simulated ECUs/Virya Controller CAN File 08082024/BMS/TX/PDUs/BMS01/sigStateOfCharge ==
  ISignal Value : Subsystem
  _sigStateOfCharge_ : BusCreator  Inputs=1
  sigStateOfCharge : Outport
  wires:
  _sigStateOfCharge_/1 -> sigStateOfCharge/1  "sigStateOfCharge"
  ISignal Value/1(ISignal Value) -> _sigStateOfCharge_/1  "ISignal Value"

== system DriveSystemControl/Bus Configuration (1) - In/Simulated ECUs/Virya Controller CAN File 08082024/BMS/TX/PDUs/BMS02/sigBatteryCurrent ==
  ISignal Value : Subsystem
  _sigBatteryCurrent_ : BusCreator  Inputs=1
  sigBatteryCurrent : Outport
  wires:
  _sigBatteryCurrent_/1 -> sigBatteryCurrent/1  "sigBatteryCurrent"
  ISignal Value/1(ISignal Value) -> _sigBatteryCurrent_/1  "ISignal Value"

== system DriveSystemControl/Bus Configuration (1) - In/Simulated ECUs/Virya Controller CAN File 08082024/BMS/TX/PDUs/BMS02/sigDriveCurrentLimit ==
  ISignal Value : Subsystem
  _sigDriveCurrentLimit_ : BusCreator  Inputs=1
  sigDriveCurrentLimit : Outport
  wires:
  _sigDriveCurrentLimit_/1 -> sigDriveCurrentLimit/1  "sigDriveCurrentLimit"
  ISignal Value/1(ISignal Value) -> _sigDriveCurrentLimit_/1  "ISignal Value"

== system DriveSystemControl/Bus Configuration (1) - In/Simulated ECUs/Virya Controller CAN File 08082024/BMS/TX/PDUs/BMS02/sigRegenCurrentLimit ==
  ISignal Value : Subsystem
  _sigRegenCurrentLimit_ : BusCreator  Inputs=1
  sigRegenCurrentLimit : Outport
  wires:
  _sigRegenCurrentLimit_/1 -> sigRegenCurrentLimit/1  "sigRegenCurrentLimit"
  ISignal Value/1(ISignal Value) -> _sigRegenCurrentLimit_/1  "ISignal Value"

== system DriveSystemControl/Bus Configuration (1) - In/Simulated ECUs/Virya Controller CAN File 08082024/BMS/TX/PDUs/BMS02/sigVehicleModeRequest ==
  ISignal Value : Subsystem
  _sigVehicleModeRequest_ : BusCreator  Inputs=1
  sigVehicleModeRequest : Outport
  wires:
  _sigVehicleModeRequest_/1 -> sigVehicleModeRequest/1  "sigVehicleModeRequest"
  ISignal Value/1(ISignal Value) -> _sigVehicleModeRequest_/1  "ISignal Value"

== system DriveSystemControl/Bus Configuration (1) - In/Simulated ECUs/Virya Controller CAN File 08082024/TCU/TX/PDUs/MainController/CCU_heartBeat ==
  ISignal Value : Subsystem
  _CCU_heartBeat_ : BusCreator  Inputs=1
  CCU_heartBeat : Outport
  wires:
  _CCU_heartBeat_/1 -> CCU_heartBeat/1  "CCU_heartBeat"
  ISignal Value/1(ISignal Value) -> _CCU_heartBeat_/1  "ISignal Value"

== system DriveSystemControl/Bus Configuration (1) - In/Simulated ECUs/Virya Controller CAN File 08082024/TCU/TX/PDUs/MainController/notUsed ==
  ISignal Value : Subsystem
  _notUsed_ : BusCreator  Inputs=1
  notUsed : Outport
  wires:
  _notUsed_/1 -> notUsed/1  "notUsed"
  ISignal Value/1(ISignal Value) -> _notUsed_/1  "ISignal Value"

== system DriveSystemControl/Bus Configuration (1) - In/Simulated ECUs/Virya Controller CAN File 08082024/TCU/TX/PDUs/MainController/setAutoParkBreak ==
  ISignal Value : Subsystem
  _setAutoParkBreak_ : BusCreator  Inputs=1
  setAutoParkBreak : Outport
  wires:
  _setAutoParkBreak_/1 -> setAutoParkBreak/1  "setAutoParkBreak"
  ISignal Value/1(ISignal Value) -> _setAutoParkBreak_/1  "ISignal Value"

== system DriveSystemControl/Bus Configuration (1) - In/Simulated ECUs/Virya Controller CAN File 08082024/TCU/TX/PDUs/MainController/setBreake ==
  ISignal Value : Subsystem
  _setBreake_ : BusCreator  Inputs=1
  setBreake : Outport
  wires:
  _setBreake_/1 -> setBreake/1  "setBreake"
  ISignal Value/1(ISignal Value) -> _setBreake_/1  "ISignal Value"

== system DriveSystemControl/Bus Configuration (1) - In/Simulated ECUs/Virya Controller CAN File 08082024/TCU/TX/PDUs/MainController/setDirection ==
  ISignal Value : Subsystem
  _setDirection_ : BusCreator  Inputs=1
  setDirection : Outport
  wires:
  _setDirection_/1 -> setDirection/1  "setDirection"
  ISignal Value/1(ISignal Value) -> _setDirection_/1  "ISignal Value"

== system DriveSystemControl/Bus Configuration (1) - In/Simulated ECUs/Virya Controller CAN File 08082024/TCU/TX/PDUs/MainController/setDriveMode ==
  ISignal Value : Subsystem
  _setDriveMode_ : BusCreator  Inputs=1
  setDriveMode : Outport
  wires:
  _setDriveMode_/1 -> setDriveMode/1  "setDriveMode"
  ISignal Value/1(ISignal Value) -> _setDriveMode_/1  "ISignal Value"

== system DriveSystemControl/Bus Configuration (1) - In/Simulated ECUs/Virya Controller CAN File 08082024/TCU/TX/PDUs/MainController/setVelocity ==
  ISignal Value : Subsystem
  _setVelocity_ : BusCreator  Inputs=1
  setVelocity : Outport
  wires:
  _setVelocity_/1 -> setVelocity/1  "setVelocity"
  ISignal Value/1(ISignal Value) -> _setVelocity_/1  "ISignal Value"

== system DriveSystemControl/Bus Configuration (1) - In/Simulated ECUs/Virya Controller CAN File 08082024/TCU/TX/PDUs/MainController/steeringPower ==
  ISignal Value : Subsystem
  _steeringPower_ : BusCreator  Inputs=1
  steeringPower : Outport
  wires:
  _steeringPower_/1 -> steeringPower/1  "steeringPower"
  ISignal Value/1(ISignal Value) -> _steeringPower_/1  "ISignal Value"

== system DriveSystemControl/Bus Configuration (1) - In/Simulated ECUs/Virya Controller CAN File 08082024/TCU/TX/PDUs/TCU01/sigBrake ==
  ISignal Value : Subsystem
  _sigBrake_ : BusCreator  Inputs=1
  sigBrake : Outport
  wires:
  _sigBrake_/1 -> sigBrake/1  "sigBrake"
  ISignal Value/1(ISignal Value) -> _sigBrake_/1  "ISignal Value"

== system DriveSystemControl/Bus Configuration (1) - In/Simulated ECUs/Virya Controller CAN File 08082024/TCU/TX/PDUs/TCU01/sigControllerTemperature ==
  ISignal Value : Subsystem
  _sigControllerTemperature_ : BusCreator  Inputs=1
  sigControllerTemperature : Outport
  wires:
  _sigControllerTemperature_/1 -> sigControllerTemperature/1  "sigControllerTemperature"
  ISignal Value/1(ISignal Value) -> _sigControllerTemperature_/1  "ISignal Value"

== system DriveSystemControl/Bus Configuration (1) - In/Simulated ECUs/Virya Controller CAN File 08082024/TCU/TX/PDUs/TCU01/sigDriveMode ==
  ISignal Value : Subsystem
  _sigDriveMode_ : BusCreator  Inputs=1
  sigDriveMode : Outport
  wires:
  _sigDriveMode_/1 -> sigDriveMode/1  "sigDriveMode"
  ISignal Value/1(ISignal Value) -> _sigDriveMode_/1  "ISignal Value"

== system DriveSystemControl/Bus Configuration (1) - In/Simulated ECUs/Virya Controller CAN File 08082024/TCU/TX/PDUs/TCU01/sigMotorTemperature ==
  ISignal Value : Subsystem
  _sigMotorTemperature_ : BusCreator  Inputs=1
  sigMotorTemperature : Outport
  wires:
  _sigMotorTemperature_/1 -> sigMotorTemperature/1  "sigMotorTemperature"
  ISignal Value/1(ISignal Value) -> _sigMotorTemperature_/1  "ISignal Value"

== system DriveSystemControl/Bus Configuration (1) - In/Simulated ECUs/Virya Controller CAN File 08082024/TCU/TX/PDUs/TCU01/sigRMSCurrent ==
  ISignal Value : Subsystem
  _sigRMSCurrent_ : BusCreator  Inputs=1
  sigRMSCurrent : Outport
  wires:
  _sigRMSCurrent_/1 -> sigRMSCurrent/1  "sigRMSCurrent"
  ISignal Value/1(ISignal Value) -> _sigRMSCurrent_/1  "ISignal Value"

== system DriveSystemControl/Bus Configuration (1) - In/Simulated ECUs/Virya Controller CAN File 08082024/TCU/TX/PDUs/TCU01/sigSpeed ==
  ISignal Value : Subsystem
  _sigSpeed_ : BusCreator  Inputs=1
  sigSpeed : Outport
  wires:
  _sigSpeed_/1 -> sigSpeed/1  "sigSpeed"
  ISignal Value/1(ISignal Value) -> _sigSpeed_/1  "ISignal Value"

== system DriveSystemControl/Bus Configuration (1) - In/Simulated ECUs/Virya Controller CAN File 08082024/TCU/TX/PDUs/TCU01/sigThrottle ==
  ISignal Value : Subsystem
  _sigThrottle_ : BusCreator  Inputs=1
  sigThrottle : Outport
  wires:
  _sigThrottle_/1 -> sigThrottle/1  "sigThrottle"
  ISignal Value/1(ISignal Value) -> _sigThrottle_/1  "ISignal Value"

== system DriveSystemControl/Bus Configuration (1) - In/Simulated ECUs/Virya Controller CAN File 08082024/TCU/TX/PDUs/TCU02/sigCapacitorVoltage ==
  ISignal Value : Subsystem
  _sigCapacitorVoltage_ : BusCreator  Inputs=1
  sigCapacitorVoltage : Outport
  wires:
  _sigCapacitorVoltage_/1 -> sigCapacitorVoltage/1  "sigCapacitorVoltage"
  ISignal Value/1(ISignal Value) -> _sigCapacitorVoltage_/1  "ISignal Value"

== system DriveSystemControl/Bus Configuration (1) - In/Simulated ECUs/Virya Controller CAN File 08082024/TCU/TX/PDUs/TCU02/sigMotorRPM ==
  ISignal Value : Subsystem
  _sigMotorRPM_ : BusCreator  Inputs=1
  sigMotorRPM : Outport
  wires:
  _sigMotorRPM_/1 -> sigMotorRPM/1  "sigMotorRPM"
  ISignal Value/1(ISignal Value) -> _sigMotorRPM_/1  "ISignal Value"

== system DriveSystemControl/Bus Configuration (1) - In/Simulated ECUs/Virya Controller CAN File 08082024/TCU/TX/PDUs/TCU02/sigOdometer ==
  ISignal Value : Subsystem
  _sigOdometer_ : BusCreator  Inputs=1
  sigOdometer : Outport
  wires:
  _sigOdometer_/1 -> sigOdometer/1  "sigOdometer"
  ISignal Value/1(ISignal Value) -> _sigOdometer_/1  "ISignal Value"

== system DriveSystemControl/Bus Configuration (1) - In/Simulated ECUs/Virya Controller CAN File 08082024/TCU/TX/PDUs/TCU03/Controller_CompleteFaults ==
  ISignal Value : Subsystem
  _Controller_CompleteFaults_ : BusCreator  Inputs=1
  Controller_CompleteFaults : Outport
  wires:
  _Controller_CompleteFaults_/1 -> Controller_CompleteFaults/1  "Controller_CompleteFaults"
  ISignal Value/1(ISignal Value) -> _Controller_CompleteFaults_/1  "ISignal Value"

== system DriveSystemControl/Bus Configuration (1) - In/Simulated ECUs/Virya Controller CAN File 08082024/TCU/TX/PDUs/TCU03/sig5VSupplyFailure ==
  ISignal Value : Subsystem
  _sig5VSupplyFailure_ : BusCreator  Inputs=1
  sig5VSupplyFailure : Outport
  wires:
  _sig5VSupplyFailure_/1 -> sig5VSupplyFailure/1  "sig5VSupplyFailure"
  ISignal Value/1(ISignal Value) -> _sig5VSupplyFailure_/1  "ISignal Value"

== system DriveSystemControl/Bus Configuration (1) - In/Simulated ECUs/Virya Controller CAN File 08082024/TCU/TX/PDUs/TCU03/sigBPosOvervoltageCutback ==
  ISignal Value : Subsystem
  _sigBPosOvervoltageCutback_ : BusCreator  Inputs=1
  sigBPosOvervoltageCutback : Outport
  wires:
  _sigBPosOvervoltageCutback_/1 -> sigBPosOvervoltageCutback/1  "sigBPosOvervoltageCutback"
  ISignal Value/1(ISignal Value) -> _sigBPosOvervoltageCutback_/1  "ISignal Value"
